simulink model "VisionSystem"  (R2024b)
settings: Solver=ode3  StartTime=0  StopTime=TFinal  FixedStep=Ts  RelTol=1e-3  EnableMultiTasking=on
model workspace (MAT data in the model file):
  CIRCLE_PTS = [19 19 19]
  ZEROS = [0 0 0 0 0 0 0 0 0 0 0 0 ... (1444 elements, 38x38)]
undefined symbols (not defined in the file or in its folder): codertarget, gray, Ts
libraries: visiontextngfix x1
settings Model: ExtModeTrigDuration=80  Creator=The MathWorks, Inc.  LastModifiedBy=fears
settings SolverCC: AlgebraicLoopSolver=TrustRegion
settings DataIOCC: LimitDataPoints=on  SaveFormat=StructureWithTime  ReturnWorkspaceOutputs=off
settings OptimizationCC: BlockReduction=off  EnhancedBackFolding=on  PassReuseOutputArgsThreshold=0  MaxStackSize=64  OptimizeBlockOrder=speed  DifferentSizesBufferReuse=on  OptimizationCustomize=off
settings DebuggingCC: AlgebraicLoopMsg=none  ParameterPrecisionLossMsg=none  ParameterTunabilityLossMsg=error  BusObjectLabelMismatch=error  PregeneratedLibrarySubsystemCodeDiagnostic=none  SFUnexpectedBacktrackingDiag=warning  SFNoUnconditionalDefaultTransitionDiag=warning  SFExecutionAtInitializationDiag=none  ArithmeticOperatorsInVariantConditions=warning
settings HardwareCC: ProdBitPerPointer=32  ProdBitPerSizeT=32  ProdBitPerPtrDiffT=32  ProdLargestAtomicInteger=Long  ProdWordSize=32  ProdHWDeviceType=ARM Compatible->ARM 9  UseEmbeddedCoderFeatures=off  UseSimulinkCoderFeatures=off
settings ModelReferenceCC: EnableRefExpFcnMdlSchedulingChecks=on  ModelReferenceNumInstancesAllowed=Single  PropagateSignalLabelsOutOfModel=off
settings SFSimCC: SimUseLocalCustomCode=off  MATLABDynamicMemAlloc=off  CustomCodeUndefinedFunction=UseInterfaceOnly
settings RTWCC: Description=Embedded Coder  SystemTargetFile=ert.tlc  HardwareBoard=PARROT Mambo  TemplateMakefile=ert_default_tmf  RTWUseLocalCustomCode=off  Toolchain=Sourcery G++ Lite GNU Toolchain for Drones  GPUComputeCapability=3.5  DLArmComputeVersion=19.05
settings CodeAppCC: ForceParamTrailComments=on  MaxIdLength=63  OperatorAnnotations=on
settings ERTTargetCC: ERTCustomFileBanners=off  MatFileLogging=on  SupportContinuousTime=on  SupportNonInlinedSFcns=on  RemoveResetFunc=off  ModelStepFunctionPrototypeControlCompliant=off  InlinedParameterPlacement=Hierarchical  DynamicArrayContainerType=coder::array
settings ConfigComp: CovMetricSettings=dw  CovSaveCumulativeToWorkspaceVar=on  CovSaveSingleToWorkspaceVar=on  CovExternalEMLEnable=off  CovSFcnEnable=off

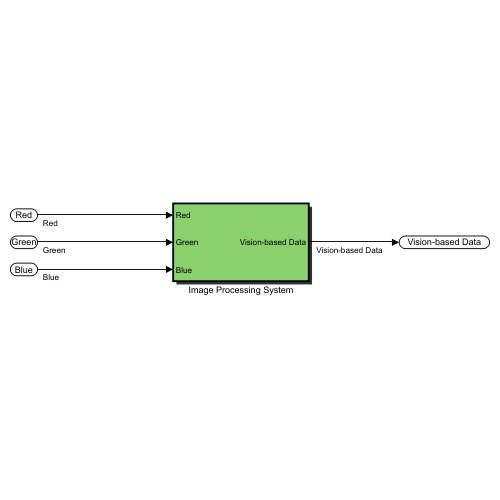
[thumbnail: Simulink's stored preview of the top-level diagram]
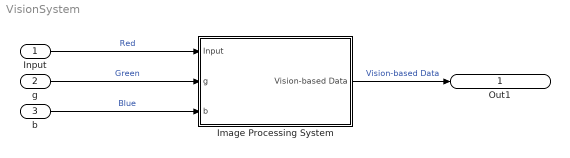
== system VisionSystem ==
  Input : Inport
  g : Inport  Port=2
  b : Inport  Port=3
  Image Processing System : Subsystem  Tag=IP_SUB  InitFcn=codertarget.parrot.internal.ipSubsystemCallback(gcb);  TreatAsAtomicUnit=on  SystemSampleTime=40*Ts  RTWFcnName=ImageFunction
      settings: RTWSystemCode=Inline  RTWFcnNameOpts=User specified
  Out1 : Outport
  wires:
  Image Processing System/1(Vision-based Data) -> Out1/1  "Vision-based Data"
  Input/1 -> Image Processing System/1(Input)  "Red"
  g/1 -> Image Processing System/2(g)  "Green"
  b/1 -> Image Processing System/3(b)  "Blue"

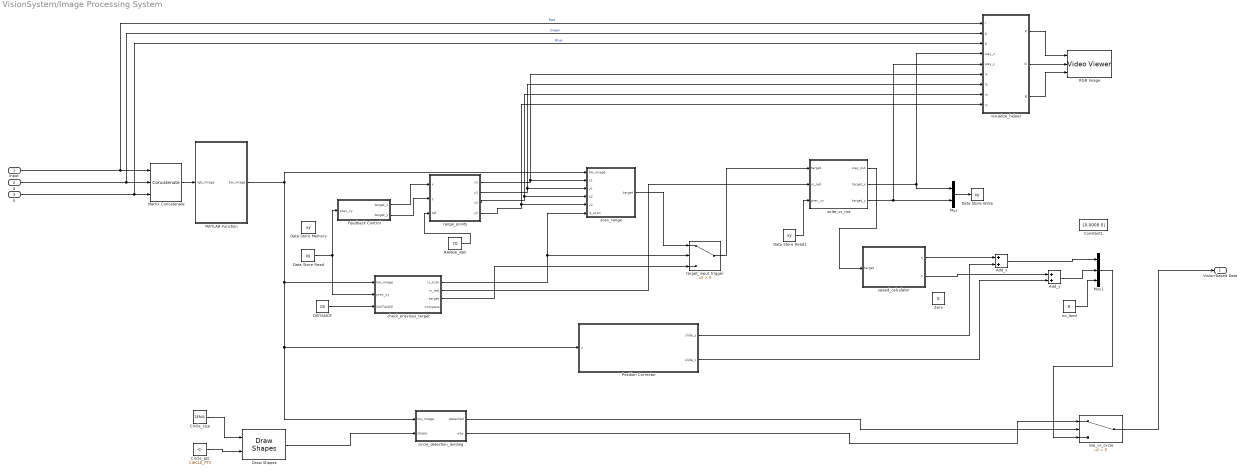
== system VisionSystem/Image Processing System ==
  Input : Inport
  g : Inport  Port=2
  b : Inport  Port=3
  Add_x : Sum
  Add_y : Sum
  Circle_pts : Constant  Value=CIRCLE_PTS
  Circle_size : Constant  Value=ZEROS
  Constant1 : Constant  Value=[0.0008 0]
  DISTANCE : Constant  Value=16
  Data Store Memory : DataStoreMemory  DataStoreName=xy  ReadBeforeWriteMsg=warning  WriteAfterWriteMsg=warning  WriteAfterReadMsg=warning  InitialValue=[0 0]  ShowAdditionalParam=off
  Data Store Read : DataStoreRead  DataStoreName=xy  IndexOptions=Index vector (dialog)  Indices=1  OutputSizes=1
  Data Store Read1 : DataStoreRead  DataStoreName=xy  IndexOptions=Index vector (dialog)  Indices=1  OutputSizes=1
  Data Store Write : DataStoreWrite  DataStoreName=xy  IndexOptions=Index vector (dialog)  Indices=1  OutputSizes=1
  Draw Shapes : visiontextngfix/Draw Shapes  shape=Circles  fill=on  lineWidth=1  fillClrSource=Specify via dialog  display=White  intensity=200  color=[200 255 100]  opacity=1  viewport=Entire image  antialiasing=off  inType=Obsolete  imagePorts=One multidimensional signal  roundingMode=Floor  overflowMode=off  memoryMode=Specify word length  memoryWordLength=16  prodOutputMode=Binary point scaling  prodOutputWordLength=32  prodOutputFracLength=14  memoryFracLength=15
  Feedback Control : MATLAB Function  TreatAsAtomicUnit=on
  MATLAB Function : MATLAB Function  TreatAsAtomicUnit=on
  Matrix Concatenate : Concatenate  NumInputs=3  Mode=Multidimensional array  ConcatenateDimension=3
  Mux : Mux  Inputs=2
  Mux1 : Mux  Inputs=3
  Position Corrector : Subsystem
  RANGE_REF : Constant  Value=70
  RGB Image : VideoViewer  imagePorts=separate color signals  colormapValue=gray(256)  FigPos=[883 1126 730 527]
  Zero : Constant  Value=0  OutDataTypeStr=Inherit: Inherit via back propagation
  check_previous_target : MATLAB Function  TreatAsAtomicUnit=on
  circle_detection_landing : MATLAB Function  TreatAsAtomicUnit=on
  line_or_circle : Switch  Criteria=u2 > Threshold  SaturateOnIntegerOverflow=off  InputSameDT=off
  no_land : Constant  Value=0
  range_points : MATLAB Function  TreatAsAtomicUnit=on
  scan_range : MATLAB Function  TreatAsAtomicUnit=on
  speed_calculator : MATLAB Function  TreatAsAtomicUnit=on
  target_input_trigger : Switch  Criteria=u2 > Threshold  SaturateOnIntegerOverflow=off  InputSameDT=off
  visualize_helper : MATLAB Function  TreatAsAtomicUnit=on
  write_or_not : MATLAB Function  TreatAsAtomicUnit=on
  Vision-based Data : Outport  VectorParamsAs1DForOutWhenUnconnected=off
  wires:
  b/1 -> visualize_helper/3(b), Matrix Concatenate/3  "Blue"
  Input/1 -> Matrix Concatenate/1, visualize_helper/1(r)  "Red"
  g/1 -> visualize_helper/2(g), Matrix Concatenate/2  "Green"
  MATLAB Function/1(bw_image) -> scan_range/1(bw_image), Position Corrector/1(u), circle_detection_landing/1(bw_image), check_previous_target/1(bw_image)
  speed_calculator/1(X) -> Add_x/1
  RANGE_REF/1 -> range_points/3(ref)
  Mux/1 -> Data Store Write/1
  visualize_helper/1(R) -> RGB Image/1
  visualize_helper/2(G) -> RGB Image/2
  visualize_helper/3(B) -> RGB Image/3
  Add_x/1 -> Mux1/1
  Add_y/1 -> Mux1/2
  speed_calculator/2(Y) -> Add_y/1
  Data Store Read/1 -> Feedback Control/1(prev_xy), check_previous_target/2(prev_xy)
  DISTANCE/1 -> check_previous_target/3(DISTANCE)
  Feedback Control/1(target_x) -> range_points/1(x)
  Feedback Control/2(target_y) -> range_points/2(y)
  range_points/1(x1) -> scan_range/2(x1), visualize_helper/6(lx)
  range_points/2(y1) -> scan_range/3(y1), visualize_helper/7(ly)
  range_points/3(x2) -> scan_range/4(x2), visualize_helper/8(rx)
  range_points/4(y2) -> scan_range/5(y2), visualize_helper/9(ry)
  write_or_not/2(target_x) -> Mux/1, visualize_helper/4(way_x)
  write_or_not/3(target_y) -> Mux/2, visualize_helper/5(way_y)
  target_input_trigger/1 -> write_or_not/1(target)
  write_or_not/1(way_out) -> speed_calculator/1(target)
  check_previous_target/2(in_red) -> write_or_not/2(in_red)
  Mux1/1 -> line_or_circle/3
  line_or_circle/1 -> Vision-based Data/1
  circle_detection_landing/1(detected) -> line_or_circle/2
  circle_detection_landing/2(way) -> line_or_circle/1
  no_land/1 -> Mux1/3
  check_previous_target/1(is_scan) -> scan_range/6(is_scan), target_input_trigger/2
  check_previous_target/3(target) -> target_input_trigger/3
  scan_range/1(target) -> target_input_trigger/1
  Data Store Read1/1 -> write_or_not/3(prev_xy)
  Matrix Concatenate/1 -> MATLAB Function/1(rgb_image)
  Draw Shapes/1 -> circle_detection_landing/2(shape)
  Circle_pts/1 -> Draw Shapes/2
  Circle_size/1 -> Draw Shapes/1
  Position Corrector/1(slide_y) -> Add_x/2
  Position Corrector/2(slide_x) -> Add_y/2

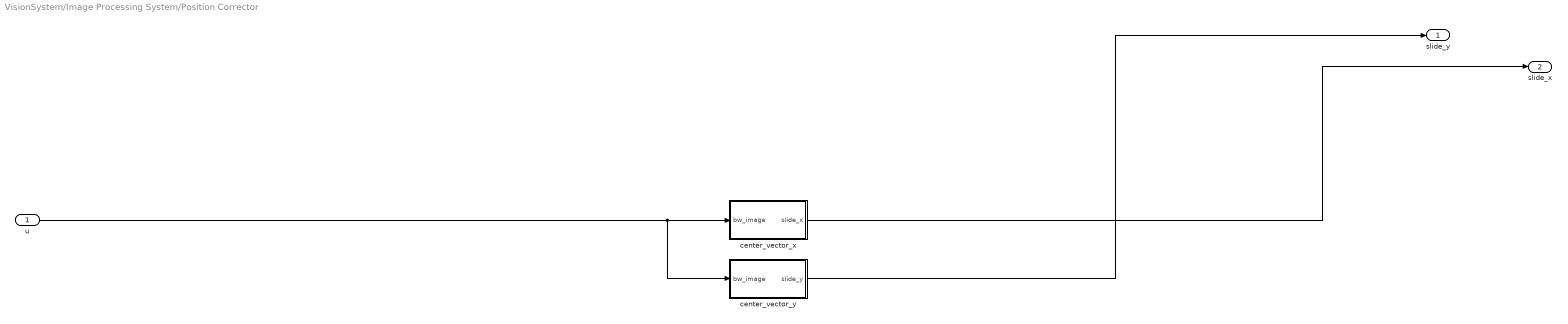
== system VisionSystem/Image Processing System/Position Corrector ==
  u : Inport
  center_vector_x : MATLAB Function  TreatAsAtomicUnit=on
  center_vector_y : MATLAB Function  TreatAsAtomicUnit=on
  slide_y : Outport
  slide_x : Outport  Port=2
  wires:
  u/1 -> center_vector_x/1(bw_image), center_vector_y/1(bw_image)
  center_vector_y/1(slide_y) -> slide_y/1
  center_vector_x/1(slide_x) -> slide_x/1

== matlab function VisionSystem/Image Processing System/visualize_helper ==
  data: r input; R output; g input; b input; way_x input; way_y input; G output; B output; lx input; ly input; rx input; ry input
function [R,G,B] = fcn(r,g,b, way_x, way_y,  lx,ly, rx,ry)

% completely unnecessary block for algorithm, just for visualize

r(60,80) = 255; g(60,80) = 255; b(60,80) = 255;

if way_x >= 1 && way_y >= 1 && way_x <= 120 && way_y <= 160


% -----------------------------------------------
    x1 = 60; y1 = 80;  x2 = way_x;   y2 = way_y;
    swapepd = 0;
    if abs(y2 - y1) > abs(x2 - x1)
        %disp('[swapped] dy bigger')
        swapepd = 1;
        [x1,y1] = deal(y1,x1);
        [x2,y2] = deal(y2,x2);
        xk = 1; yk = 1;
        if (x2 < x1) xk = -1; end
        if (y2 < y1) yk = -1; end
    else
        xk = -1; yk = -1;
        if (x2 > x1) xk = 1; end
        if (y2 > y1) yk = 1; end

    end
    dy = abs(y2-y1);
    dx = abs(x2-x1);
    % --------------------------------------
    m = 2 * dy;
    slope_error = m - 2*dx;
  
    y = y1;
    for x = x1:xk:x2
        if swapepd == 1
            r(y,x) = 255; g(y,x) = 255; b(y,x) = 255;
        else
            r(x,y) = 255; g(x,y) = 255; b(x,y) = 255;
        end
        
   
        slope_error = slope_error + m;
        if (slope_error > 0)
            y = y + yk;
            slope_error = slope_error - 2 * dx;
        end
    end
end




% --------------------------------------------
x1 = 60; y1 = 80; x2 = lx; y2 = ly;
    swapepd = 0;
    if abs(y2 - y1) > abs(x2 - x1)
        %disp('[swapped] dy bigger')
        swapepd = 1;
        [x1,y1] = deal(y1,x1);
        [x2,y2] = deal(y2,x2);
        xk = 1; yk = 1;
        if (x2 < x1) xk = -1; end
        if (y2 < y1) yk = -1; end
    else
        xk = -1; yk = -1;
        if (x2 > x1) xk = 1; end
        if (y2 > y1) yk = 1; end

    end
    dy = abs(y2-y1);
    dx = abs(x2-x1);
    % --------------------------------------
    m = 2 * dy;
    slope_error = m - 2*dx;
  
    y = y1;
    for x = x1:xk:x2
        if swapepd == 1
            g(y,x) = 255;
        else
            g(x,y) = 255;
        end
        
   
        slope_error = slope_error + m;
        if (slope_error > 0)
            y = y + yk;
            slope_error = slope_error - 2 * dx;
        end
    end
% -----------------------------------------

    x1 = 60; y1 = 80; x2 = rx; y2 = ry;
    swapepd = 0;
    if abs(y2 - y1) >= abs(x2 - x1)
        %disp('[swapped] dy bigger')
        swapepd = 1;
        [x1,y1] = deal(y1,x1);
        [x2,y2] = deal(y2,x2);
        xk = 1; yk = 1;
        if (x2 < x1) xk = -1; end
        if (y2 < y1) yk = -1; end
    else
        xk = -1; yk = -1;
        if (x2 > x1) xk = 1; end
        if (y2 > y1) yk = 1; end

    end
    dy = abs(y2-y1);
    dx = abs(x2-x1);
    % --------------------------------------
    m = 2 * dy;
    slope_error = m - 2*dx;
  
    y = y1;
    for x = x1:xk:x2
        if swapepd == 1
            if x <1 break; end
            g(y,x) = 255;
        else
            g(x,y) = 255;
        end
        
   
        slope_error = slope_error + m;
        if (slope_error > 0)
            y = y + yk;
            slope_error = slope_error - 2 * dx;
        end
    end

b(40:80, 60:90) = 200;
R = r;
G = g;
B = b;
end

== matlab function VisionSystem/Image Processing System/write_or_not ==
  data: target input; way_out output; in_red input; prev_xy input; target_x output; target_y output
function [way_out, target_x, target_y] = fcn(target, in_red, prev_xy)

x = target(1);
y = target(2);
speed = target(3);

if in_red
    X = x;   Y = y;
    target_x = x;  target_y = y;%output as a valid target
else
    X = x;  Y = y; 
    target_x = prev_xy(1);  
    target_y = prev_xy(2);%dont move and start a new loop
end

way_out = [X Y speed];

%fprintf('X = %f | Y = %f\n', target_x, target_y);
end

== matlab function VisionSystem/Image Processing System/MATLAB Function ==
  data: rgb_image input; bw_image output
function bw_image = red_detection_binarize(rgb_image)
    %  RGB To HSV
    hsv_image = rgb2hsv(rgb_image);

    % HSV Parameters_red
    h_min = 0;    % Min Hue 
    h_max = 0.1;  % Max Hue
    s_min = 0.3;  % Min Saturation
    s_max = 1;    % Max Saturation
    v_min = 0.1;  % Min Value
    v_max = 1;    % Max Value

    % Mask 
    mask1 = (hsv_image(:,:,1) >= h_min & hsv_image(:,:,1) <= h_max) & ...
            (hsv_image(:,:,2) >= s_min & hsv_image(:,:,2) <= s_max) & ...
            (hsv_image(:,:,3) >= v_min & hsv_image(:,:,3) <= v_max);
    mask2 = (hsv_image(:,:,1) >= 0.9 & hsv_image(:,:,1) <= 1) & ...
            (hsv_image(:,:,2) >= s_min & hsv_image(:,:,2) <= s_max) & ...
            (hsv_image(:,:,3) >= v_min & hsv_image(:,:,3) <= v_max);

    % Mask Sum
    red_mask = mask1 | mask2;

    % Keep red  mask, set others black
    masked_rgb = rgb_image;
    masked_rgb(repmat(~red_mask, [1, 1, 3])) = 0;

    % Mask To Grey
    gray_image = rgb2gray(masked_rgb);

    % Grey To Binizaration
    level = graythresh(gray_image);       % Calculate threshold
    bw_image = imbinarize(gray_image, level); 

    % Noise Filter
    %u = bwareaopen(u, 50);
end

== matlab function VisionSystem/Image Processing System/speed_calculator ==
  data: target input; X output; Y output
function [X,Y] = fcn(target)

x = target(1);
y = target(2);
speed = target(3);

if speed == 100
    speed = 200;
elseif speed < 60
    speed = 60;
end


X = (60-x) / 10000000 * speed;
Y = (y-80) / 10000000 * speed;


%fprintf(' --- speed: %f | ', speed); fprintf('vectors: X=%.5f | Y=%.5f\n', X, Y);

end

== matlab function VisionSystem/Image Processing System/Feedback Control ==
  data: target_x output; prev_xy input; target_y output
function [target_x, target_y] = fcn(prev_xy)

    x = prev_xy(1);
    y = prev_xy(2);
    
    if x == 0 || y == 0 %initial satate
        target_x = 0;
        target_y = 0;
    else
        target_x = 60 + (60 - x) + 1; %1--120
        target_y = 80 + (80 - y) + 1; %2--159
    end

    %fprintf('opposite: %.0f %.0f -> %.0f %.0f\n', x, y, way_x, way_y);
end

== matlab function VisionSystem/Image Processing System/Position Corrector/center_vector_x ==
  data: bw_image input; slide_x output
function slide_x = fcn(bw_image) 
%input:bw_image,bw_image
%output:slide_x,x direction velocity

%initialize centerpoint
c1 = 60; 
c2 = 80;
left_p = 0;
right_p = 0;
center = bw_image(c1, c2);
compare = ~center;

%find left bound
for i = c2:-1:60 % <---  look left
    if bw_image(c1, i) == compare
        left_p = i;
        break
    end
end

%find right bound
for i = c2:100 % --->   look right
    if bw_image(c1, i) == compare
        right_p = i;
        break
    end
end

slide_x = 0;
if left_p ~= 0 && right_p ~= 0 % in line
    if center == 1
        vr = right_p - c2;  % length right 
        vl = c2 - left_p;   % length left
        diff = vr-vl;%calculate diff to center
        slide_x = get_speed(diff) * 20;%back to center
    end
end
end

function T = get_speed(t)

if t > 0 %too left
    if t < 1 %slowly adjust position when diif is small
        T = 0.000001;
    elseif t < 5
        T = 0.000002;
    elseif t < 10
        T = 0.000003;
    elseif t < 15
        T = 0.000004;
    elseif t < 20
        T = 0.000005;
    else
        T = 0.000006;
    end
else %too right
    if t < -20
        T = -0.000006;
    elseif t < -15
        T = -0.000005;
    elseif t < -10
        T = -0.000004;
    elseif t < -5
        T = -0.000003;
    elseif t < -1
        T = -0.000002;
    else
        T = -0.000001;
    end
end

end

== matlab function VisionSystem/Image Processing System/range_points ==
  data: x input; x1 output; y input; ref input; y1 output; x2 output; y2 output
function [x1,y1, x2,y2] = get_range_points(x,y, ref)

% x1, y1 are left
% x2, y2 are right 
% according to center-to-edge vector.

W = edge_number(x,y);

if W == 1%up bound
    y1 = y - ref;%To left
    if y1 < 1
        x1 = x - y1;%become left
        y1 = 1;
    else
        x1 = x;
    end

    y2 = y + ref;%To right
    if y2 > 160
        x2 = y2-160;%become right
        y2 = 160;
    else
        x2 = x;
    end
elseif W == 2%left bound
    x1 = x + ref;
    if x1 > 120
        y1 = x1 - 120;
        x1 = 120;
    else
        y1 = y;
    end

    x2 = x - ref;
    if x2 < 1
        y2 = abs(x2) + 1;
        x2 = 1;
    else
        y2 = y;
    end
elseif W == 4%right bound
    x1 = x - ref;
    if x1 < 1
        y1 = 160 + x1;
        x1 = 1;
    else
        y1 = 160;
    end

    x2 = x + ref;
    if x2 > 120
        y2 = 160 - (x2 - 120);
        x2 = 120;
    else
        y2 = y;
    end
elseif W == 3%down bound
    y1 = y + ref;%159+70=229
    if y1 > 160
        x1 = 120 - (y1-160);%51
        y1 = 160;
    else
        x1 = x;
    end

    y2 = y - ref;%89
    if y2 < 1
        x2 = 120 + y2;
        y2 = 1;
    else
        x2 = x;%120
    end
else %initial state and rescan
    x1 = 1; y1 = 1;
    x2 = 1; y2 = 2;
end

%fprintf('range_points: %.0f-%.0f  to  %.0f-%.0f\n', x1,y1, x2,y2);

end

== matlab function VisionSystem/Image Processing System/Position Corrector/center_vector_y ==
  data: bw_image input; slide_y output
function slide_y = fcn(bw_image)
c1 = 60; 
c2 = 80;
up_p = 0;
down_p = 0;
center = bw_image(c1,c2);
compare = ~center;
for i = c1:-1:40 % look up
    if bw_image(i, c2) == compare
        up_p = i;
        break
    end
end
for i = c1:80 % look down
    if bw_image(i, c2) == compare
        down_p = i;
        break
    end
end
slide_y = 0;
if up_p ~= 0 && down_p ~= 0  % in line
    if center == 1
        vu = down_p - c1;  %length up
        vd = c1 - up_p;    %length down
        diff = vd-vu;
        
        slide_y = get_speed(diff) * 20;
    end
end

end
function T = get_speed(t)

if t > 0
    if t <= 1
        T = 0.000001;
    elseif t < 5
        T = 0.000002;
    elseif t < 10
        T = 0.000003;
    elseif t < 15
        T = 0.000005;
    elseif t < 20
        T = 0.000005;
    else
        T = 0.000005;
    end
else
    if t < -20
        T = -0.000005;
    elseif t < -15
        T = -0.000005;
    elseif t < -10
        T = -0.000004;
    elseif t <= -5
        T = -0.000003;
    elseif t < -1
        T = -0.000002;
    else
        T = -0.000001;
    end
end
end

== matlab function VisionSystem/Image Processing System/scan_range ==
  data: target output; bw_image input; x1 input; y1 input; x2 input; y2 input; is_scan input
function target  = scan_range(bw_image, x1,y1, x2,y2, is_scan)

target_x = 1;
target_y = 2;
speed = 0;
in_red_line = bw_image(60, 80);


persistent prev_endless_x;
persistent prev_endless_y;

if is_scan
    if in_red_line == 1  % ------ inside red-line ------
    
        t = 0;
        mx = 0;

        mx_endless_x = [0 0];
        mx_endless_y = [0 0];
        mx_t = [0 0];

        last_endless = false;
        index_of_endless = 0;
        
        w1 = edge_number(x1,y1);
        xi = x1;  yi = y1; k = 1;
        
        if w1 == 1 || w1 == 4
            k = -1;
        end
        
        
        while xi ~= x2 || yi ~= y2 %iterate through all pixel between point1 and point2
            returned = line_drawer(60, 80, xi, yi, bw_image, 0);%return value if a pixel on the line between (60,80) and iterate point is 0(have end)

            if returned == 0 % if endless: every pixel value is 1

                if last_endless == false
                    last_endless = true;
                    index_of_endless = index_of_endless + 1;
                end
                if index_of_endless > 2
                    break;
                end
                
                mx_endless_x(index_of_endless) = mx_endless_x(index_of_endless) + xi;
                mx_endless_y(index_of_endless) = mx_endless_y(index_of_endless) + yi;
                mx_t(index_of_endless) = mx_t(index_of_endless) + 1;

            else%path has end one pixel on line is 0
                last_endless = false;
                if returned > mx
                    mx = returned;
                    target_x = xi; % output end point 
                    target_y = yi;
                    t = 1;
                end
            end

            % İteration x for each y(row by row)
            temp_w = edge_number(xi, yi); 
            if temp_w == 1 || temp_w == 3
                yi = yi + k;
            else
                xi = xi + k;
            end
            if xi < 1%clamping boundary
                yi = 159; xi = 1; k = -1;
            elseif xi > 120
                xi = 120; yi = 2; k = 1;
            elseif yi < 1
                yi = 1; xi = 2; k = 1;
            elseif yi > 160
                yi = 160; xi = 119; k = -1;
            end
        end % while end


        if index_of_endless == 1 % ---------- 1 endless ------------
            %fprintf('only one endless!\n');
            target_x = mx_endless_x(1);
            target_y = mx_endless_y(1);
            t = mx_t(1);

            target_x = round(target_x/t);
            target_y = round(target_y/t);
            [target_x, target_y] = nearest_edge(target_x, target_y);

            prev_endless_x = 60 + (60 - target_x) + 1;
            prev_endless_y = 80 + (80 - target_y) + 1;

        elseif index_of_endless == 2 % ---------- 2 endless ------------
            
            if isempty(prev_endless_x)
                target_x = mx_endless_x(1);
                target_y = mx_endless_y(1);
                t = mx_t(1);
    
                target_x = round(target_x/t);
                target_y = round(target_y/t);
                [target_x, target_y] = nearest_edge(target_x, target_y);
    
                prev_endless_x = 60 + (60 - target_x) + 1;
                prev_endless_y = 80 + (80 - target_y) + 1;
            else
                mid_calculated = [0 0; 0 0];
                for i = 1:2
                    x = mx_endless_x(i);
                    y = mx_endless_y(i);
                    t = mx_t(i);

                    x = round(x/t);
                    y = round(y/t);
                    
                    [x,y] = nearest_edge(x, y);
                    
                    mid_calculated(i, 1) = x;
                    mid_calculated(i, 2) = y;
                end
                %fprintf('calculated = %.0f %.0f  | %.0f %.0f\n', ...
                %    mid_calculated(1,1), mid_calculated(1,2), ...
                %    mid_calculated(2,1), mid_calculated(2,2));

                diff_x1 = prev_endless_x-mid_calculated(1,1);
                diff_y1 = prev_endless_y-mid_calculated(1,2);
                diff_x2 = prev_endless_x-mid_calculated(2,1);
                diff_y2 = prev_endless_y-mid_calculated(2,2);
                diff1 = sqrt(diff_x1*diff_x1 + diff_y1*diff_y1);
                diff2 = sqrt(diff_x2*diff_x2 + diff_y2*diff_y2);

                if diff1 > diff2
                    target_x = mid_calculated(1,1);
                    target_y = mid_calculated(1,2);
                else
                    target_x = mid_calculated(2,1);
                    target_y = mid_calculated(2,2);
                end
                
                prev_endless_x = 60 + (60 - target_x) + 1;
                prev_endless_y = 80 + (80 - target_y) + 1;
                
            end
        else % ---------- NO endless ------------
            speed = mx;
        end

        

    else % ----------------- outside red line ----------------------
        x1 = 2; y1 = 1;
        x2 = 1; y2 = 1;
        
        ENDLESS = 100;
        mn = ENDLESS;
        w1 = edge_number(x1,y1);
        xi = x1;  yi = y1;  k = 1;
        if w1 == 1 || w1 == 4
            k = -1;
        end
        
        while xi ~= x2 || yi ~= y2
            returned = line_drawer(60, 80, xi, yi, bw_image, 1);
    
            if returned > 0 && returned < mn
                mn = returned;
                target_x = xi;
                target_y = yi;
            end
    
            % İteration
            temp_w = edge_number(xi, yi);
            if temp_w == 1 || temp_w == 3
                yi = yi + k;
            else
                xi = xi + k;
            end
            if xi < 1
                yi = 159; xi = 1; k = -1;
            elseif xi > 120
                xi = 120; yi = 2; k = 1;
            elseif yi < 1
                yi = 1; xi = 2; k = 1;
            elseif yi > 160
                yi = 160; xi = 119; k = -1;
            end
        end % while
        
        speed = 100;
        if mn < 60
            speed = 60;
        end
    end % if redline end

end % is_scan

target = [target_x, target_y, speed];

end % function end

== matlab function VisionSystem/Image Processing System/check_previous_target ==
  data: bw_image input; is_scan output; in_red output; prev_xy input; DISTANCE input; target output; compare output
function [is_scan, in_red, target,compare]  = fcn(bw_image, prev_xy, DISTANCE)

prev_x = prev_xy(1);
prev_y = prev_xy(2);

in_red = bw_image(60, 80);
compare = ~in_red;

is_scan = 0;
target_x = 1;
target_y = 1;
speed = 0;

if prev_x == 0 || prev_y == 0 %scan when prev_coordinates unvalid
    is_scan = 1;
else 
    if bw_image(prev_x, prev_y) == 1 %prev_coordinates in red

        %continue upload new coordinats
        [ref_x, ref_y] = middle_point_of_endless_line(bw_image, prev_x, prev_y);

        target_x = prev_x + ref_x;
        target_y = prev_y + ref_y;
        
        %boundary limit. make path in image
        if target_y > 160
            if target_x == 120 
                target_x = 120 - mod(target_y, 160);
            elseif target_x == 1 
                target_x = mod(target_y, 160);
            end
            target_y = 160;
            
        elseif target_y < 1
            if target_x == 120 
                target_x = 120 - abs(target_y);
            elseif target_x == 1 
                target_x = abs(target_y); 
            end
            target_y = 1;
            
        elseif target_x < 1
            if target_y == 160
                target_y = 160 - abs(target_x);
            elseif target_y == 1
                target_y = abs(target_x);
            end
            target_x = 1;
            
        elseif target_x > 120
            if target_y == 160
                target_y = 160 - (target_x - 120);
            elseif target_y == 1
                target_y = target_x - 120;
            end
            target_x = 120;
        end

        %{
        if target_x < 1   target_x = 1;   end
        if target_x > 120 target_x = 120; end
        if target_y < 1   target_y = 1;   end
        if target_y > 160 target_y = 160; end
        %}
        speed = 100;

    else %target not in red
        
        % endless dissappeared ----------------------------
        if in_red
            distance = line_drawer(60, 80, prev_x, prev_y, bw_image, compare);
            if distance < DISTANCE
                is_scan = 1;
                speed = 0;
            else
                speed = distance;
            end
            
            target_x = prev_x;
            target_y = prev_y;
        else
            is_scan = 1;
            target_x = prev_x;
            target_y = prev_y;
            speed = 40;
        end

    end
end
target = [target_x, target_y, speed];

end % func end



function [ref_x, ref_y] = middle_point_of_endless_line(bw_image, target_x, target_y)

w = edge_number(target_x, target_y);

if w == 1 || w == 3

    % to right
    iter_y = target_y;
    iter_x = target_x;
    plus_or_minus = 1;
    x_or_y = 0; % 0:y   1:x
    distance = 0;

    while bw_image(iter_x, iter_y) == 1
        if x_or_y == 0
            iter_y = iter_y + plus_or_minus;
        else
            iter_x = iter_x + plus_or_minus;
        end
        distance = distance + 1;
        
        if iter_y > 160
            iter_y = 160;
            x_or_y = 1;
            if iter_x == 120
                plus_or_minus = -1;
            elseif iter_x == 1
                plus_or_minus = 1;
            end
        end
        if iter_x < 1
            break;
        elseif iter_x > 120
            break;
        end
    end
    right = distance;

    % to left
    iter_y = target_y;
    iter_x = target_x;
    plus_or_minus = -1;
    x_or_y = 0; % 0:y   1:x
    distance = 0;
    
    while bw_image(iter_x, iter_y) == 1
        if x_or_y == 0
            iter_y = iter_y + plus_or_minus;
        else
            iter_x = iter_x + plus_or_minus;
        end
        distance = distance + 1;

        if iter_y < 1
            iter_y = 1;
            x_or_y = 1;
            if iter_x == 120
                plus_or_minus = -1;
            elseif iter_x == 1
                plus_or_minus = 1;
            end
        end
        if iter_x < 1
            break
        elseif iter_x > 120
            break
        end
    end
    left = distance;
    
    
    ref_x = 0;
    diff = right - left;
    
    if abs(diff) >= 7 && abs(diff) < 25
        ref_y = round(diff/2);
    else
        ref_y = 0;
    end

else % ------------------------- 2 & 4 --------------------------
    % to up
    iter_x = target_x;
    iter_y = target_y;
    plus_or_minus = -1;
    x_or_y = 1; % 0:y   1:x
    distance = 0;
    while bw_image(iter_x, iter_y) == 1
        if x_or_y == 0
            iter_y = iter_y + plus_or_minus;
        else
            iter_x = iter_x + plus_or_minus;
        end
        distance = distance + 1;

        if iter_x < 1
            iter_x = 1;
            x_or_y = 0;
            if iter_y == 1
                plus_or_minus = 1;
            elseif iter_y == 160
                plus_or_minus = -1;
            end
        end
        if iter_y > 160
            break
        elseif iter_y < 1
            break
        end
    end
    up = distance;

    % to down
    iter_x = target_x;
    iter_y = target_y;
    plus_or_minus = 1;
    x_or_y = 1; % 0:y   1:x
    distance = 0;
    while bw_image(iter_x, iter_y) == 1
        if x_or_y == 0
            iter_y = iter_y + plus_or_minus;
        else
            iter_x = iter_x + plus_or_minus;
        end
        distance = distance + 1;
        if iter_x > 120
            x_or_y = 0;
            iter_x = 120;
            if iter_y == 1
                plus_or_minus = 1;
            elseif iter_y == 160
                plus_or_minus = -1;
            end
        end
        if iter_y > 160
            break;
        elseif iter_y < 1
            break;
        end
    end
    down = distance;

    diff = down - up;

    ref_y = 0;
    if abs(diff) >= 7 && abs(diff) < 25
        ref_x = round(diff/2);
    else
        ref_x = 0;
    end
end

end

== matlab function VisionSystem/Image Processing System/circle_detection_landing ==
  data: bw_image input; detected output; way output; shape input
function [detected, way] = fcn(bw_image, shape)

persistent landing;
if isempty(landing)
    landing = 0;
end

detected = 0;
way = [0 0 0];
land = 0;

%landing order
if landing == 1
    way = [0 0 1];
    detected = 1;

else
    [total_pixel, cord_x, cord_y] = detect_circle(bw_image, shape);
    
    if total_pixel >= 1350%circle detection parameters
        detected = 1;
        center_x = cord_x + 19;%shape parameters
        center_y = cord_y + 19;%shape parameters
    
        %Image boundary limit
        if center_x > 120
            center_x = 120;
        end
        if center_y > 160
            center_y = 160;
        end
        
        %landing order limit
        dif_x = round(60 - center_x);
        dif_y = round(center_y - 80);
        %calculate 
        dist = sqrt(dif_x * dif_x + dif_y * dif_y);
    
        fprintf(' #### CIRCLE - centers: %3.1f %3.1f | dist: %3.1f\n', ...
            center_x, center_y, dist);
    
        if dist < 15
            land = 1;
            landing = 1;
        end
        way_x = dif_x / 130000;
        way_y = dif_y / 130000;
        way = [way_x way_y land];
    end

end

end

function [total_pixel, cord_x, cord_y] = detect_circle(bw_image, shape)

%  total_pixel: sum of number of pixel
%       cord_x: row coordinate of bw_image
%       cord_y: column coordinate of bw_image

[circle_size_x, circle_size_y] = size(shape);
R = 120;  C = 160;

total_pixel = 0;
cord_x = 0;
cord_y = 0;

%circle detection, a slide window
for i = 1:(R - circle_size_x)
    for j = 1:(C - circle_size_y)
        section = bw_image(i:i+circle_size_x-1, j:j+circle_size_y-1);
        result = sum(~xor(section, shape), 'all');
        if result > total_pixel
            total_pixel = result;
            cord_x = i;
            cord_y = j;
        end
    end

end
end
